simulink model "Anti_Windup"  (R2025a)
settings: Solver=VariableStepAuto  StartTime=0.0  StopTime=10.0  RelTol=1e-3
settings Model: Creator=xing2  LastModifiedBy=xing2

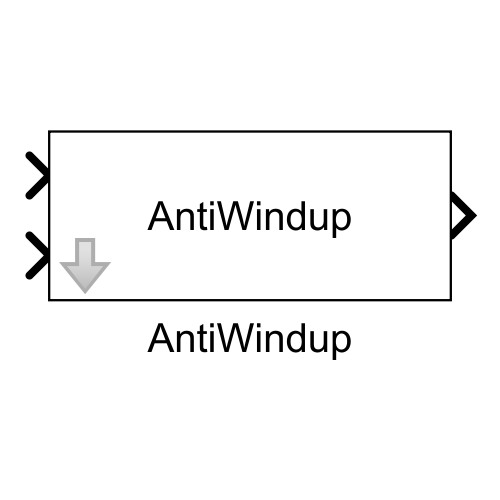
[thumbnail: Simulink's stored preview of the top-level diagram]
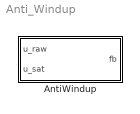
== system Anti_Windup ==
  AntiWindup : Subsystem  mask{Kaw=1}
      mask help: Anti-Windup: Kaw*(u_sat-u_raw)
      mask Display: disp('AntiWindup');

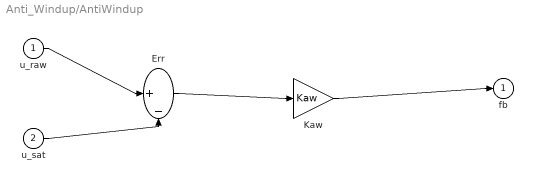
== system Anti_Windup/AntiWindup ==
  u_raw : Inport
  u_sat : Inport  Port=2
  Err : Sum  Inputs=|+-
  Kaw : Gain  Gain=Kaw
  fb : Outport
  wires:
  u_raw/1 -> Err/1
  u_sat/1 -> Err/2
  Err/1 -> Kaw/1
  Kaw/1 -> fb/1
